simulink model "Motor_Revised_MOSFET_CHB"  (R2017b)
settings: Solver=ode45  StartTime=0.0  StopTime=1800  RelTol=1e-3  EnableMultiTasking=on
undefined symbols (not defined in the file or in its folder): vehicle_weight
libraries: powerlib x5
settings Model: PauseTimes=1154  Creator=fengqi.chang  LastModifiedBy=fengqi.chang
settings DataIOCC: LimitDataPoints=on  SaveFormat=Array
settings OptimizationCC: LifeSpan=inf
settings DebuggingCC: SolverPrmCheckMsg=warning  SFUnexpectedBacktrackingDiag=warning  SFNoUnconditionalDefaultTransitionDiag=warning  SFExecutionAtInitializationDiag=none
settings HardwareCC: ProdBitPerPointer=32  ProdBitPerSizeT=32  ProdBitPerPtrDiffT=32  ProdLargestAtomicFloat=None  ProdIntDivRoundTo=Undefined  ProdEndianess=Unspecified  ProdWordSize=32  ProdHWDeviceType=32-bit Generic
settings ModelReferenceCC: PropagateSignalLabelsOutOfModel=off
settings CodeAppCC: StateflowObjectComments=on
settings GRTTargetCC: TargetLangStandard=C89/C90 (ANSI)  GeneratePreprocessorConditionals=Disable all
settings ConfigComp: CovMetricSettings=dw  CovHtmlReporting=on  CovSaveCumulativeToWorkspaceVar=on  CovSaveSingleToWorkspaceVar=on  CovExternalEMLEnable=off  CovSFcnEnable=off
settings SimscapeCC: SimscapeNormalizeSystem=off

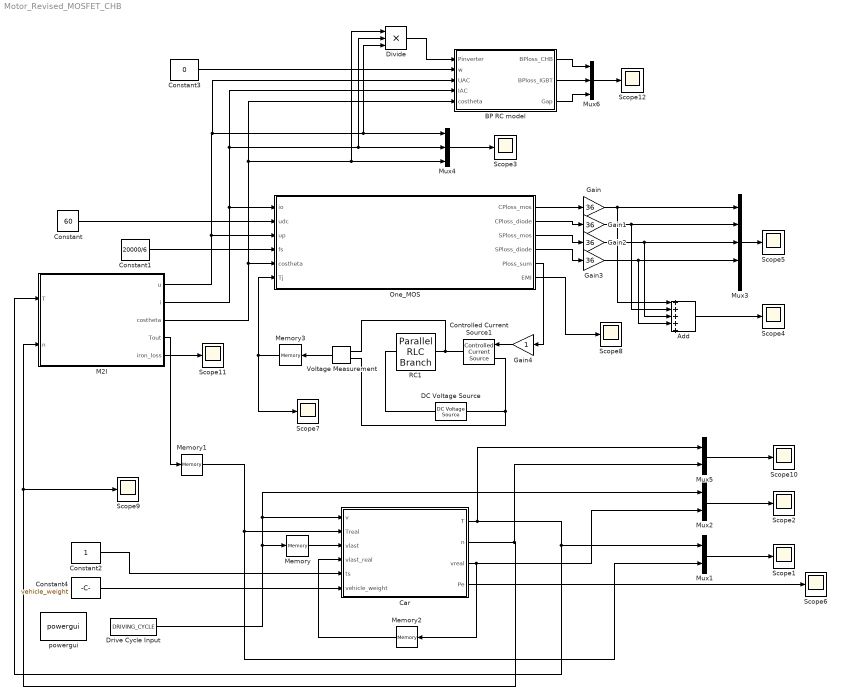
== system Motor_Revised_MOSFET_CHB ==
  Add : Sum  Inputs=+++++
  BP RC model : MATLAB Function  TreatAsAtomicUnit=on
  Car : MATLAB Function  TreatAsAtomicUnit=on
  Constant : Constant  Value=60
  Constant1 : Constant  Value=20000/6
  Constant2 : Constant
  Constant3 : Constant  Value=0
  Constant4 : Constant  Value=vehicle_weight
  Controlled Current Source1 : powerlib/Electrical Sources/Controlled Current Source  Initialize=on  Source_Type=DC  Amplitude=0  Phase=0  Frequency=0  Measurements=None
  DC Voltage Source : powerlib/Electrical Sources/DC Voltage Source  Amplitude=30  Measurements=None
  Divide : Product  Inputs=***
  Drive Cycle Input : FromWorkspace  VariableName=DRIVING_CYCLE  SampleTime=1  OutputAfterFinalValue=Setting to zero
  Gain{,1..3} (4 alike) : Gain  Gain=36
  Gain4 : Gain
  M2I : MATLAB Function  TreatAsAtomicUnit=on
  Memory : Memory  InheritSampleTime=on
  Memory1 : Memory  InheritSampleTime=on
  Memory2 : Memory  InheritSampleTime=on
  Memory3 : Memory  InitialCondition=25  InheritSampleTime=on
  Mux1 : Mux  Inputs=2
  Mux2 : Mux  Inputs=2
  Mux3 : Mux  Inputs=5
  Mux4 : Mux  Inputs=3
  Mux5 : Mux  Inputs=2
  Mux6 : Mux  Inputs=3
  One_MOS : MATLAB Function  TreatAsAtomicUnit=on
  RC1 : powerlib/Elements/Parallel RLC Branch  LConnTagsString=a  RConnTagsString=__new0  BranchType=R  Resistance=0.5  Inductance=1e-3  SetiL0=off  InitialCurrent=0  Capacitance=0  Setx0=on  InitialVoltage=0  Measurements=None
  Scope{1..12} (12 alike) : Scope
  Voltage Measurement : powerlib/Measurements/Voltage Measurement  PhasorSimulation=off  OutputType=Complex  PSBequivalent=0
  powergui : powerlib/powergui  Priority=1  SimulationMode=Discrete  SampleTime=1  frequency=60  Iterations=50  frequencyindice=0  Pbase=100e6  ErrMax=1e-4  UnitsV=kV  UnitsW=MW  buscounter=0  FunctionMessages=off  echomessages=off  EnableUseOfTLC=off  CurrentSourceSwitches=off  DisableSnubberDevices=off  DisableRonSwitches=off  DisableVfSwitches=off  DisplayEquations=off  SolverType=Backward Euler  Interpol=off  ExternalGateDelay=off  methode=off  Ts=100  x0status=blocks  SPID=off  SwTol=0  HookPort=off  RestoreLinks=warning  ResistiveCurrentMeasurement=off  Frange=[0:2:500]  Ylog=off  Xlog=on  ShowGrid=off  save=off  variable=ZData  structure=0  ZoomFFT=off  StartTime=0.0  cycles=1  DisplayStyle=1  fundamental=60  FreqAxis=off  MaxFrequency=1000  frequencyindicesteady=1  RmsSteady=1  display=off
  wires:
  Car/1(T) -> Mux5/1, M2I/1(T), Mux1/1
  Car/2(n) -> Mux5/2, Scope9/1, M2I/2(n)
  Car/3(vreal) -> Memory2/1, Mux2/2
  M2I/3(costheta) -> BP RC model/5(costheta), Divide/1, Mux4/3, One_MOS/5(costheta)
  Constant/1 -> One_MOS/2(udc)
  Constant1/1 -> One_MOS/4(fs)
  One_MOS/1(CPloss_mos) -> Gain/1
  One_MOS/2(CPloss_diode) -> Gain1/1
  One_MOS/3(SPloss_mos) -> Gain2/1
  One_MOS/4(SPloss_diode) -> Gain3/1
  Constant2/1 -> Car/5(ts)
  Gain/1 -> Add/1, Mux3/1
  Gain1/1 -> Add/2, Mux3/2
  Gain2/1 -> Mux3/3, Add/3
  Gain3/1 -> Add/4, Mux3/4
  Drive Cycle Input/1 -> Memory/1, Car/1(v), Mux2/1
  M2I/4(Tout) -> Memory1/1
  M2I/1(u) -> BP RC model/3(UAC), Divide/3, Mux4/1, One_MOS/3(up)
  Mux1/1 -> Scope1/1
  Memory1/1 -> Mux1/2, Car/2(Treal)
  Mux2/1 -> Scope2/1
  Memory/1 -> Car/3(vlast)
  Memory2/1 -> Car/4(vlast_real)
  M2I/2(i) -> BP RC model/4(IAC), Divide/2, Mux4/2, One_MOS/1(io)
  Car/4(Pe) -> Scope6/1
  Add/1 -> Scope4/1
  Mux3/1 -> Scope5/1
  Mux4/1 -> Scope3/1
  Voltage Measurement/1 -> Memory3/1
  Memory3/1 -> Scope7/1, One_MOS/6(Tj)
  One_MOS/5(Ploss_sum) -> Gain4/1
  Divide/1 -> BP RC model/1(Pinverter)
  One_MOS/6(EMI) -> Scope8/1
  Gain4/1 -> Controlled Current Source1/1
  Constant3/1 -> BP RC model/2(w)
  Mux5/1 -> Scope10/1
  M2I/5(iron_loss) -> Scope11/1
  Constant4/1 -> Car/6(vehicle_weight)
  Mux6/1 -> Scope12/1
  BP RC model/1(BPloss_CHB) -> Mux6/1
  BP RC model/2(BPloss_IGBT) -> Mux6/2
  BP RC model/3(Gap) -> Mux6/3
  connections:
  Controlled Current Source1/RConn1 -- Voltage Measurement/LConn1 -- RC1/RConn1
  DC Voltage Source/RConn1 -- RC1/LConn1
  DC Voltage Source/LConn1 -- Voltage Measurement/LConn2 -- Controlled Current Source1/LConn1

== matlab function Motor_Revised_MOSFET_CHB/M2I ==
  data: T input; n input; u output; i output; costheta output; Tout output; iron_loss output
function [u,i,costheta,Tout,iron_loss] = PMSM2Inverter_Pcalc(T,n)
%%%%%%%%%%%%%%%%%%%%%%%Variable Table%%%%%%%%%%%%%%%%%%%%%%%%%%%%
%u          SQRT(3/2)*peak value of the output phase voltage from inverter    (V)
%i          SQRT(3/2)*peak value of the output phase current from inverter    (A)
%costheta   power factor required by the motor                      (none)
%T          torque required by the car                              (Nm)
%n          rotation speed of the motor required by the car         (rpm)
%%%%%%%%%%%%%%%%%%%%%%%%%%%%%%%%%%%%%%%%%%%%%%%%%%%%%%%%%%%%%%%%%
%%created in 2016 02 01 10 29
%%the model defines the interface of motor to inverter, which calculates 
%%the current, voltage as well as the power factor required by a motor.  
%%this model ignores the electrical transient status of the motor, but the
%%error caused is unclear yet.
%%this model is only valid for induction motor. For more complex ones,
%%model should be revised. 
%%%%%%%%%%%%%%%%%%%%%%%%Parameters%%%%%%%%%%%%%%%%%%%%%%%%%%%%%%%
Lq=8.0955e-5;
Ld=7.0955e-5;
p=6;%pair of polars
R=0.009;%resistor on stator, ohm%%%
psyr=0.05345836;%rotor permanent flux, Vs%%%
irate=450;%rated stator current, A, phase rms value
urate=160.1;%rated stator voltage, V, phase rms value
Prate=125000;%rated machinery power, W,
%%%%%%%%%%%%%%%%%%input preparation%%%%%%%%%%%%%%%%%%%%
wr=n*p/60*2*pi;
isq=T/p/psyr;
isd=0;
usd=-Lq*isq*wr+R*isd;
usq=(Ld*isd+psyr)*wr+R*isq;

i=sqrt(isq*isq+isd*isd);
u=sqrt(usq*usq+usd*usd);
costheta=(usd*isd+usq*isq)/u/i;%cos(atan(usq/usd)-atan(isq/isd));
Tout=T;
%%%%%%%%%%%%%if flux weakening required%%%%%%%%%%%%%%%%
if(u>(urate*sqrt(3)))
    if(abs(n*T*2*pi/60)>=Prate)
        Tout=Prate/(n/60*2*pi);
    else
        Tout=T;
    end
    psy_l=0;
    psy_h=psyr;
    psy_iter=(psy_l+psy_h)/2;
    u_iter=u;
    while(abs(urate*sqrt(3)-u_iter)>1)%iteration to calculate the right psy to reach urate
        isd=(psy_iter-psyr)/Ld;
        isq=T/(p*psyr+p*(Ld-Lq)*isd);
        usd=-Lq*isq*wr+R*isd;
        usq=(Ld*isd+psyr)*wr+R*isq;
        u=sqrt(usq*usq+usd*usd);
        u_iter=u;
        if(u_iter>urate*sqrt(3))
            psy_h=psy_iter;
            psy_iter=0.5*(psy_l+psy_h);
        else
            psy_l=psy_iter;
            psy_iter=0.5*(psy_l+psy_h);
        end
    end
    
end
i=sqrt(isq*isq+isd*isd);
u=sqrt(usq*usq+usd*usd);
costheta=(usd*isd+usq*isq)/u/i;%cos(atan(usq/usd)-atan(isq/isd));
% if(i>(irate*sqrt(3)))
%     isq=isq*irate*1.414/i;%no max torque algorithm is applied
%     isd=isd*irate*1.414/i;
%     Tout=isq*p/Lr*Lm*isd*Lm;
%     wsl=Tout/p*Rr/(Lm*isd)^2;
%     wk=wsl+n*p/60*2*pi;
%     usd=Rs*isd-wk*(Ls*isq+Lm*(-isq*Lm/Lr));
%     usq=Rs*isq+wk*Ls*isd;
%     i=sqrt(isq*isq+isd*isd);%
%     u=sqrt(usq*usq+usd*usd);
% end
%iron_loss = (9.128008725474993e-06*n^2 + 0.119030169537619*n)/3.3007*(abs(T)^0.5186);
beta = [7.47991049806284e-06,-0.00164430283336243,0.152741302836017,0.945215242366288];
iron_loss = (beta(1).*n.^2 + beta(2).*n).*beta(3).*(abs(T).^beta(4));

if isnan(costheta)
    costheta=1;
end
if(n<0.1)&&(T==0)
    u=0;
    i=0;
    Tout=0;
    costheta=1;
end
if (Tout~=T)
    Tout=T;
end

== matlab function Motor_Revised_MOSFET_CHB/Car ==
  data: v input; T output; Treal input; vlast input; vlast_real input; ts input; n output; vreal output; Pe output; vehicle_weight input
function [T,n,vreal,Pe] = CarModel(v,Treal,vlast,vlast_real,ts,vehicle_weight)
%%%%%%%%%%%%%%%%%%%%%%%%%%%%varialbe table%%%%%%%%%%%%%%%%%%%%%%%%%%%%%%%%%
%variavle name      meaning,                                             unit
%a,                 acceleration order of the car,                       (m/s^2)
%v,                 speed order of the car,                              (m/s)
%T,                 torque of the motor required by the car,             (Nm)
%n,                 rotation speed of the motor,                         (rpm)
%Pe,                power of the motor required by the car,              (kW)
%a_real,            real acceleration of the car,                        (m/s^2)
%vlast,             real speed of the car in last simulation period,     (m/s)
%nlast,             real rotation speed of the motor in last period,     (rad/s)
%Treal,             real torque from motor in  last simulation period,   (Nm)
%vnext,             real speed of the car,                               (m/s)
%ts,                simulation period,                                   (s)
%%%%%%%%%%%%%%%%%%%%%%%%%%%%%%%%%%%%%%%%%%%%%%%%%%%%%%%%%%%%%%%%%%%%%%%%%%%
%%%%%%%%%%%%%%%%%%%%%%%%%%%%parameter table%%%%%%%%%%%%%%%%%%%%%%%%%%%%%%%%
m=vehicle_weight;%1443.331;%1195;%                                  mass of the car,                      (kg)
yeta_t=0.98;%                             efficiency of the transmission,       ()

i_g=9.7;%                                 transmission ratio fo the driveline,  ()
R=0.350;%                                 radius of the tyre,                   (m)
mr=106.67*R-13.179;%                      mass of the tyre,                     (kg)
Im=0.070;%                                inertia of the motor rotor,           (Kg*m^2)

%%%%%%%%%%%%%%%%%%%%%%%%%%%%%%%%%%%%%%%%%%%%%%%%%%%%%%%%%%%%%%%%%%%%%%%%%%%
a=(v-vlast)/ts;%calculate the acceleration needed in the next simulation period
%nlast=vlast/R*i_g;%calculate the real rotation speed in the last simulation period, but right now in rad/s
if (vlast==0)&&(a==0)
    T=0;
else
    T = 1/yeta_t*(105.0138054720000+6.602356610980250*(vlast+v)/2+0.260513017636277*(vlast^2+v^2)/2+m*a)/(1/R*i_g);
    %T=1/yeta_t*(G*f/1000+Cd*A*(vlast^2+v^2)/2/1631.94+sigma*m/1000*a)*1000/(1/R*i_g);%calculate the torque needed in the next simulation period
end;
if (vlast==0)&&(Treal==0)
    areal=0;
else
    areal=(Treal*1/R*i_g*yeta_t-105.0138054720000-6.602356610980250*(vlast+v)/2-0.260513017636277*(vlast^2+v^2)/2)/(m);%calculate the real acceleration using Treal provided by the last simulation period
end
if(T<=0)&&(vlast_real<=0)
    T=0;
    areal=0;
end;
vreal=vlast_real+areal*ts;%calculate the real speed in the next simulation period
n=(v+vlast)/2/R*i_g*30/pi;%calculate the real rotation speed in the next simulation period, in rpm
Pe=n*T/60*2*pi;%calculate the power needed in the next simulation period
end

== matlab function Motor_Revised_MOSFET_CHB/One_MOS ==
  data: io input; udc input; up input; fs input; CPloss_mos output; CPloss_diode output; costheta input; SPloss_mos output; SPloss_diode output; Ploss_sum output; Tj input; EMI output
%% created in 2016 03 04 13 43
%% the model defines the input and output of the loss model of one MOSFET switch
%% that is only the simplest version of an MOSFET model
%% needs further edition
function [CPloss_mos,CPloss_diode,SPloss_mos,SPloss_diode,Ploss_sum,EMI] = MOSFET_INFENEON_100N10S3(io,udc,up,fs,costheta,Tj)
%% this model is only for voltage source inverter or converter
%%%%%%%%%%%%%%%%%%%%%%%%%%%%parameter table%%%%%%%%%%%%%%%%%%%%%%%%%%%%%%%%
io=io/sqrt(3/2);
up=up/sqrt(3/2);
n=6;%paralleled number
n1=3;%series connected number
ron=0.004*((Tj-25)*0.024+1);%@25degree, @150degress is 1.98V
rc=0;%resistor on the line and connection, usually ignored
rd=0.00185;%resistor on the diode path, usually ignored
m=up/udc/n1;%modulation index
udsat=0.71;%
Qrr=380*10^(-9);%C
%udc=400;
UDrr=udc;%V
UDD=udc;%V,DC bus voltage of the module
IDon=2*io/pi/n;
RG=2.2;%gate resistor 1Ohm
Cgd1=38.49*10^(-12);%F
Cgd2=3*10^(-9);%F
UDr=15;%V
Uplateau=5.5;%V
tri=17*10^(-9)/3.5*RG;%s, current rise time
tfu=(UDD-ron*IDon)*RG*(Cgd1+Cgd2)/(UDr-Uplateau)/2;%s, voltage fall time
tru=(UDD-ron*IDon)*RG*(Cgd1+Cgd2)/(UDr+Uplateau)/2;
tfi=20*10^(-9)/3.5*RG;
Eon_mos=UDD*abs(IDon)*0.5*(tri+tfu)+Qrr*UDD;% that is only the typical value, the value is influenced by T,r_gate and Ic
Eoff_mos=UDD*abs(IDon)*0.5*(tru+tfi);%that is only the typical value, the value is influenced by T,r_gate and Ic
Eon_diode=Qrr*UDrr;%that value is usually neglected
Eoff_diode=0;%that is only the typical value, the value is influenced by T,r_gate and Ic
%%%%%%%%%%%%%%%%%%%%%%%%%%%%varialbe table%%%%%%%%%%%%%%%%%%%%%%%%%%%%%%%%%
%variavle name      meaning,                                             unit
%io,                operation current, peak value of phase current,      (A)
%up,                operation voltage, peak value of phase voltage,      (V)
%udc,               DC bus voltage,                                      (V)
%fs,                switching frequency,                                 (Hz)
%costheta,          power factor,                                        (none)
%CPloss_igbt,       conduction loss on MOSFET                            (W)
%CPloss_diode,      conduction loss on the reverse paralleled diode,     (W)
%SPloss_igbt,       switching loss on MOSFET,                            (W)
%SPloss_diode,      switching loss on the reverse paralleled diode,      (W)
%%%%%%%%%%%%%%%%%%%%%%%%%%%%%%%%%%%%%%%%%%%%%%%%%%%%%%%%%%%%%%%%%%%%%%%%%%%
%theta=acos(costheta);

if(io*ron/4>=udsat)
	CPloss_mos=io*io*ron*(1/8+m*costheta/3/pi)/n;
	CPloss_diode=io*io*rd*(1/8-m*costheta/3/pi)/n + abs(io)*udsat*(1/2/pi-m*costheta/8);
else
    CPloss_mos=(ron+rc)*io*io/4/n;
    CPloss_diode=0;
end

SPloss_mos=fs*(Eon_mos+Eoff_mos)*n;%switching loss of a half bridge
SPloss_diode=fs*(Eon_diode+Eoff_diode)*n;%switching loss of a half bridge

Ploss_sum=(CPloss_mos+CPloss_diode+SPloss_mos+SPloss_diode)/n;

didtr=IDon/tri/10^9;
didtf=IDon/tfi/10^9;
dudtr=(UDD-ron*IDon)/tru/10^9;
dudtf=(UDD-ron*IDon)/tfu/10^9;
EMI=[didtr,didtf,dudtr,dudtf];%kV/us or kA/us
if(io==0)
   SPloss_mos=0;
   SPloss_diode=0;
end

== matlab function Motor_Revised_MOSFET_CHB/BP RC model ==
  data: Pinverter input; BPloss_CHB output; w input; UAC input; IAC input; costheta input; BPloss_IGBT output; Gap output
function [BPloss_CHB, BPloss_IGBT, Gap] = BatteryPack_RC_model(Pinverter,w,UAC,IAC,costheta)
%%%%%%%%%%%%%%%%%%%%%%%%%%%%%%%%%%%%%%%
fs = 10000;%The switching frequency
C = 475 * 1e-6;%DC link capacitance
% i=(Pinverter/(series*parallel))/(upack/series);%calculate the average DC current of the battery pack in IGBT
% w=w*2;%w is the frequency of the DC side current of the CHB, i.e., double the AC current
% RC_up=complex(0.0608*6.75,0.051*6.75*w)*parallel/series;%Using the battery parameter to calculate the battery resistance
% RC_dw=complex(120,120*1.2571*w);%Using the battery parameter to calculate the battery resistance
%dividing RC_up with RC_dw, the resistance of the battery cell at the double AC frequency is obtained

%%%%%%%%%%%%%%%%%%%%%%%%%%%%%%%%%%%%%%%%
% U=i*RC_up/RC_dw;


Ibatave = abs(UAC*IAC*costheta/9/60);
%module ave current of the CHB

% Using the denoted cell, equivalent number of parallel in each CHB module
% and in the battery pack of the IGBT
par_n_CHB = 1.8;
par_n_IGBT = 2.7;
ma = abs(UAC/sqrt(1.5))/3/75;
% Modulation index, considering fully charged status
Rcell_10k = 0.6/1000;
% 10kHz resistance of the battery, according to the reference
Rcell_DC = 1.7/1000;
% DC resistance of the battery, according to the reference, according to the reference
Rcell_AC = 0.7/1000;
% AC frequency resistance of the battery, according to the reference

Ibatrms = 2*Ibatave/costheta*sqrt((1+1/3*cos(2*acos(costheta)))/pi/ma);% rms of CHB battery module current
Icellrms = Ibatrms/par_n_CHB;% rms of cell current
Icell_ave = abs(UAC*IAC*costheta/360/par_n_IGBT);% average current

Ibat_10k_RMS = 2*Ibatave/costheta*sqrt(1/24/pi/ma*(24-6*pi*ma+(8-3*pi*ma)*cos(2*acos(costheta))))/par_n_CHB;%10kHz current ripple RMS value per cell, in CHB
Ibat_ACf_RMS = sqrt(Icellrms^2 - Ibat_10k_RMS^2 - Icell_ave^2);% AC frequency current ripple RMS value per cell, in CHB

rV = (-1.09*ma^2 + 0.74*ma);
deltaV = 1/fs*IAC/sqrt(3/2)/C*rV/96/sqrt(2);
deltaI = deltaV/Rcell_10k/3;
% RMS value of the current ripple on the DC link of the IGBT inverter

PDC_CHB = (Icell_ave)^2*Rcell_DC;%battery loss per cell caused by DC current in the CHB
PAC_CHB = Rcell_10k*(Ibat_10k_RMS)^2 + Rcell_AC*Ibat_ACf_RMS^2;%battery loss per cell caused by ripples in the CHB
PDC_IGBT = (Icell_ave)^2*Rcell_DC;%battery loss per cell  caused by DC current in the IGBT inverter
PAC_IGBT = Rcell_10k*(deltaI^2);%battery loss per cell caused by ripples in the IGBT inverter
APP = (PDC_CHB + PAC_CHB - PDC_IGBT - PAC_IGBT)*par_n_IGBT*96;%Multiply the total number of cells
APP1 = (PDC_CHB + PAC_CHB)*par_n_IGBT*96;%Total battery loss of the CHB, waiting to identify if NAN is encountered
APP2 = (PDC_IGBT + PAC_IGBT)*par_n_IGBT*96;%Total battery loss of the CHB, waiting to identify if NAN is encountered

if isnan(APP)
    APP = 0;
    APP1 = 0;
    APP2 = 0;
elseif((UAC<10*sqrt(1.5)))
%      APP = 0;
end
BPloss_CHB = APP1;
BPloss_IGBT = APP2;
Gap = APP;
